simulink model "Ejercicio7_27_03_17"  (R2013a)
settings: Solver=ode45  StartTime=0.0  StopTime=10.0  RelTol=1e-3
libraries: powerlib x11, powerlib_meascontrol x5
settings Model: Creator=Miguel  LastModifiedBy=Miguel

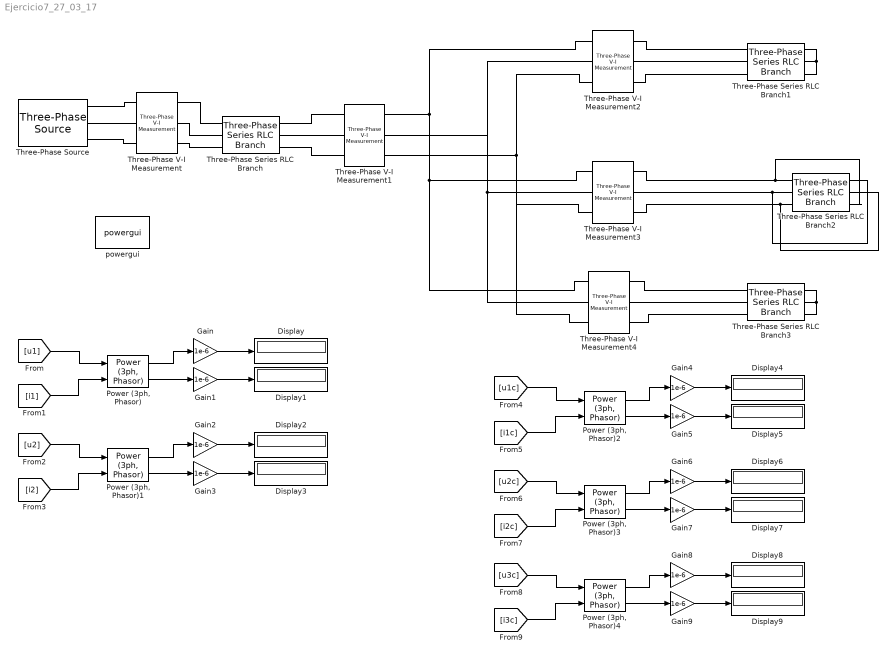
== system Ejercicio7_27_03_17 ==
  Display{,1..9} (10 alike) : Display
  Gain{,1..9} (10 alike) : Gain  Gain=1e-6
  Power (3ph, Phasor){,1..4} (5 alike) : powerlib_meascontrol/Measurements/Power (3ph, Phasor)
  Three-Phase Series RLC Branch : powerlib/Elements/Three-Phase Series RLC Branch  LConnTagsString=A|B|C  RConnTagsString=A|B|C  BranchType=RL  Resistance=1  Inductance=2/(2*pi*60)  Capacitance=1e-6  Measurements=None
  Three-Phase Series RLC Branch1 : powerlib/Elements/Three-Phase Series RLC Branch  LConnTagsString=A|B|C  RConnTagsString=A|B|C  BranchType=RL  Resistance=65  Inductance=55/(2*pi*60)  Capacitance=1e-6  Measurements=None
  Three-Phase Series RLC Branch2 : powerlib/Elements/Three-Phase Series RLC Branch  LConnTagsString=A|B|C  RConnTagsString=A|B|C  BranchType=RL  Resistance=450  Inductance=360/(2*pi*60)  Capacitance=1e-6  Measurements=None
  Three-Phase Series RLC Branch3 : powerlib/Elements/Three-Phase Series RLC Branch  LConnTagsString=A|B|C  RConnTagsString=A|B|C  BranchType=RL  Resistance=75  Inductance=60/(2*pi*60)  Capacitance=1e-6  Measurements=None
  Three-Phase V-I Measurement : powerlib/Measurements/Three-Phase V-I Measurement  VoltageMeasurement=phase-to-ground  SetLabelV=on  LabelV=u1  Vpu=off  VpuLL=off  CurrentMeasurement=yes  SetLabelI=on  LabelI=i1  Ipu=off  Pbase=100e6  Vbase=500e3  OutputType=Complex  PhasorSimulation=on  PSBequivalent=0
  Three-Phase V-I Measurement1 : powerlib/Measurements/Three-Phase V-I Measurement  VoltageMeasurement=phase-to-ground  SetLabelV=on  LabelV=u2  Vpu=off  VpuLL=off  CurrentMeasurement=yes  SetLabelI=on  LabelI=i2  Ipu=off  Pbase=100e6  Vbase=500e3  OutputType=Complex  PhasorSimulation=on  PSBequivalent=0
  Three-Phase V-I Measurement2 : powerlib/Measurements/Three-Phase V-I Measurement  VoltageMeasurement=phase-to-ground  SetLabelV=on  LabelV=u1c  Vpu=off  VpuLL=off  CurrentMeasurement=yes  SetLabelI=on  LabelI=i1c  Ipu=off  Pbase=100e6  Vbase=500e3  OutputType=Complex  PhasorSimulation=on  PSBequivalent=0
  Three-Phase V-I Measurement3 : powerlib/Measurements/Three-Phase V-I Measurement  VoltageMeasurement=phase-to-ground  SetLabelV=on  LabelV=u2c  Vpu=off  VpuLL=off  CurrentMeasurement=yes  SetLabelI=on  LabelI=i2c  Ipu=off  Pbase=100e6  Vbase=500e3  OutputType=Complex  PhasorSimulation=on  PSBequivalent=0
  Three-Phase V-I Measurement4 : powerlib/Measurements/Three-Phase V-I Measurement  VoltageMeasurement=phase-to-ground  SetLabelV=on  LabelV=u3c  Vpu=off  VpuLL=off  CurrentMeasurement=yes  SetLabelI=on  LabelI=i3c  Ipu=off  Pbase=100e6  Vbase=500e3  OutputType=Complex  PhasorSimulation=on  PSBequivalent=0
  Three-Phase Source : powerlib/Electrical Sources/Three-Phase Source  Voltage=116e3  PhaseAngle=0  Frequency=60  InternalConnection=Yg  SpecifyImpedance=off  Resistance=0  Inductance=10/(60*2*pi)  ShortCircuitLevel=100e6  BaseVoltage=116e3  XRratio=7  BusType=swing  Pref=0  Qref=0  Qmin=-inf  Qmax=inf
  powergui : powerlib/powergui  Priority=1  SimulationMode=Phasor  SolverType=Tustin  SampleTime=50e-6  frequency=60  SPID=off  DisableSnubberDevices=off  DisableRonSwitches=off  DisableVfSwitches=off  SwTol=0  Interpol=off  DisplayEquations=off  frequencyindice=60  Pbase=100e6  ErrMax=1e-4  Iterations=50  UnitsV=kV  UnitsW=MW  FunctionMessages=off  echomessages=off  HookPort=off  EnableUseOfTLC=off  x0status=blocks  RestoreLinks=warning  ResistiveCurrentMeasurement=off  Frange=[0:2:500]  Ylog=off  Xlog=on  ShowGrid=off  save=off  variable=ZData  ZoomFFT=off  StartTime=0.0  cycles=1  DisplayStyle=1  fundamental=60  FreqAxis=off  MaxFrequency=1000  frequencyindicesteady=1  RmsSteady=2  display=off  Ts=0  methode=off
  wires:
  [u1] -> "Power (3ph, Phasor)"/1
  [i1] -> "Power (3ph, Phasor)"/2
  "Power (3ph, Phasor)"/2 -> Gain1/1
  "Power (3ph, Phasor)"/1 -> Gain/1
  Gain1/1 -> Display1/1
  Gain/1 -> Display/1
  [u2] -> "Power (3ph, Phasor)1"/1
  [i2] -> "Power (3ph, Phasor)1"/2
  "Power (3ph, Phasor)1"/2 -> Gain3/1
  "Power (3ph, Phasor)1"/1 -> Gain2/1
  Gain3/1 -> Display3/1
  Gain2/1 -> Display2/1
  [u1c] -> "Power (3ph, Phasor)2"/1
  [i1c] -> "Power (3ph, Phasor)2"/2
  "Power (3ph, Phasor)2"/2 -> Gain5/1
  "Power (3ph, Phasor)2"/1 -> Gain4/1
  Gain5/1 -> Display5/1
  Gain4/1 -> Display4/1
  [u2c] -> "Power (3ph, Phasor)3"/1
  [i2c] -> "Power (3ph, Phasor)3"/2
  "Power (3ph, Phasor)3"/2 -> Gain7/1
  "Power (3ph, Phasor)3"/1 -> Gain6/1
  Gain7/1 -> Display7/1
  Gain6/1 -> Display6/1
  [u3c] -> "Power (3ph, Phasor)4"/1
  [i3c] -> "Power (3ph, Phasor)4"/2
  "Power (3ph, Phasor)4"/2 -> Gain9/1
  "Power (3ph, Phasor)4"/1 -> Gain8/1
  Gain9/1 -> Display9/1
  Gain8/1 -> Display8/1
  connections:
  Three-Phase Source/RConn1 -- Three-Phase V-I Measurement/LConn1
  Three-Phase Source/RConn2 -- Three-Phase V-I Measurement/LConn2
  Three-Phase Source/RConn3 -- Three-Phase V-I Measurement/LConn3
  Three-Phase Series RLC Branch/LConn3 -- Three-Phase V-I Measurement/RConn3
  Three-Phase V-I Measurement1/LConn1 -- Three-Phase Series RLC Branch/RConn1
  Three-Phase V-I Measurement1/LConn2 -- Three-Phase Series RLC Branch/RConn2
  Three-Phase V-I Measurement1/LConn3 -- Three-Phase Series RLC Branch/RConn3
  Three-Phase Series RLC Branch3/LConn1 -- Three-Phase V-I Measurement4/RConn1
  Three-Phase V-I Measurement2/LConn2 -- Three-Phase V-I Measurement1/RConn2 -- Three-Phase V-I Measurement4/LConn2 -- Three-Phase V-I Measurement3/LConn2
  Three-Phase V-I Measurement4/LConn3 -- Three-Phase V-I Measurement3/LConn3 -- Three-Phase V-I Measurement1/RConn3 -- Three-Phase V-I Measurement2/LConn3
  Three-Phase Series RLC Branch/LConn1 -- Three-Phase V-I Measurement/RConn1
  Three-Phase Series RLC Branch/LConn2 -- Three-Phase V-I Measurement/RConn2
  Three-Phase Series RLC Branch1/RConn1 -- Three-Phase Series RLC Branch1/RConn2 -- Three-Phase Series RLC Branch1/RConn3
  Three-Phase Series RLC Branch3/RConn1 -- Three-Phase Series RLC Branch3/RConn2 -- Three-Phase Series RLC Branch3/RConn3
  Three-Phase V-I Measurement2/RConn3 -- Three-Phase Series RLC Branch1/LConn3
  Three-Phase V-I Measurement2/RConn2 -- Three-Phase Series RLC Branch1/LConn2
  Three-Phase V-I Measurement2/RConn1 -- Three-Phase Series RLC Branch1/LConn1
  Three-Phase Series RLC Branch2/RConn2 -- Three-Phase V-I Measurement3/RConn3 -- Three-Phase Series RLC Branch2/LConn3
  Three-Phase V-I Measurement3/RConn2 -- Three-Phase Series RLC Branch2/RConn1 -- Three-Phase Series RLC Branch2/LConn2
  Three-Phase Series RLC Branch2/LConn1 -- Three-Phase Series RLC Branch2/RConn3 -- Three-Phase V-I Measurement3/RConn1
  Three-Phase V-I Measurement4/RConn2 -- Three-Phase Series RLC Branch3/LConn2
  Three-Phase V-I Measurement4/LConn1 -- Three-Phase V-I Measurement3/LConn1 -- Three-Phase V-I Measurement2/LConn1 -- Three-Phase V-I Measurement1/RConn1
  Three-Phase Series RLC Branch3/LConn3 -- Three-Phase V-I Measurement4/RConn3
